simulink model "single_phase_inverter"  (R2019b)
settings: Solver=VariableStepAuto  StartTime=0.0  StopTime=0.4  RelTol=1e-3
values from neighbouring files (symbols this model uses):
  A = [-R1/L1 0 -1/L1;      0 -R2/L2 1/L2;      1/C1 -1/C1 0]    [inverter_singlephase.m]    (also in inverter_singlephase_rpi.m)
  Ae = [-R1/L1 0 -1/L1 0 0;      0 -R2/L2 1/L2 -1/L2 0;      1/C1 -1/C1 0 0 0 ... (first row only)    [inverter_singlephase.m]    (also in inverter_singlephase_rpi.m)
  B = [1/L1 0 0]'    [inverter_singlephase.m]    (also in inverter_singlephase_rpi.m)
  Be = [1/L1 0 0 0 0]'    [inverter_singlephase.m]    (also in inverter_singlephase_rpi.m)
  C = [1 0 0; 0 0 1]    [inverter_singlephase.m]    (also in inverter_singlephase_rpi.m)
  Ce = [1 0 0 0 0; 0 0 1 0 0]    [inverter_singlephase.m]    (also in inverter_singlephase_rpi.m)
  d = 3.5e-1    (= 0.35)    [inverter_singlephase.m]    (also in inverter_singlephase_rpi.m)
  E = [0 -1/L2 0]'    [inverter_singlephase.m]    (also in inverter_singlephase_rpi.m)
  K = place(A,B,[-150*2*pi,-120*2*pi,-140*2*pi])    [inverter_singlephase.m]
  L1 = 250e-6    (= 0.00025)    [inverter_singlephase.m]    (also in inverter_singlephase_rpi.m)
  L2 = 60e-6    (= 6e-05)    [inverter_singlephase.m]    (also in inverter_singlephase_rpi.m)
  Le = place(Ae',Ce',[p1,p2,p3,p4,p5])'    [inverter_singlephase.m]
  N = -inv(C(1,:)*(A-B*K)^-1*B)    [inverter_singlephase.m]
  w = 5*w0    (= 1570.79632679)    [inverter_singlephase.m]    (also in inverter_singlephase_rpi.m)
settings Model: Creator=dbagn  LastModifiedBy=dbagn

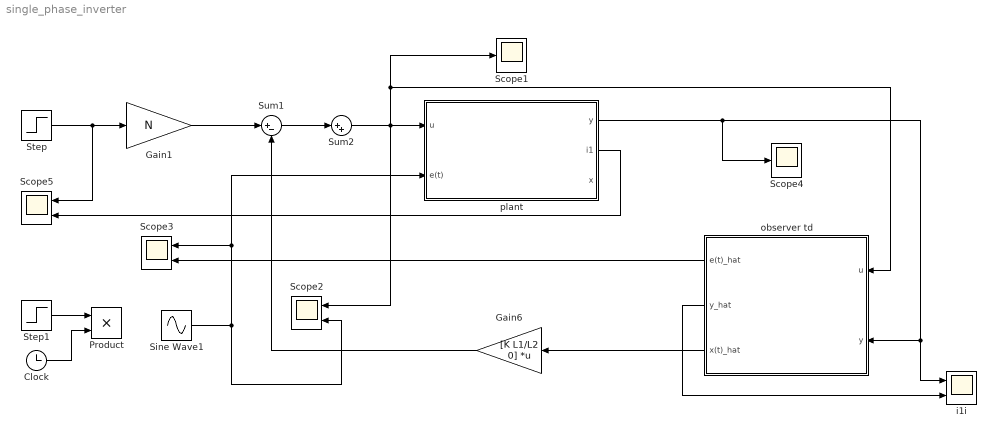
== system single_phase_inverter ==
  Clock : Clock
  Gain1 : Gain  Gain=N
  Gain6 : Gain  Gain=[K L1/L2 0]  Multiplication=Matrix(K*u)
  Product : Product
  Scope1 : Scope
  Scope2 : Scope  NumInputPorts=2
  Scope3 : Scope  NumInputPorts=2
  Scope4 : Scope
  Scope5 : Scope  NumInputPorts=2
  Sine Wave1 : Sin  Amplitude=d  Frequency=w  SampleTime=0
  Step : Step  Time=0.05  SampleTime=0
  Step1 : Step  Time=0.2  SampleTime=0
  Sum1 : Sum  Inputs=|+-
  Sum2 : Sum  Inputs=|++
  i1i : Scope  NumInputPorts=2
  observer td : Subsystem
  "plant " : Subsystem
  wires:
  observer td/2(y_hat) -> i1i/2
  "plant "/1(y) -> i1i/1, observer td/2(y), Scope4/1
  Sine Wave1/1 -> "plant "/2(e(t)), Scope3/1, Scope2/2
  observer td/1(e(t)_hat) -> Scope3/2
  "plant "/2(i1) -> Scope5/2
  Step/1 -> Gain1/1, Scope5/1
  Gain6/1 -> Sum1/2
  Gain1/1 -> Sum1/1
  Sum1/1 -> Sum2/1
  Sum2/1 -> Scope2/1, Scope1/1, observer td/1(u), "plant "/1(u)
  Step1/1 -> Product/1
  Clock/1 -> Product/2
  observer td/3(x(t)_hat) -> Gain6/1

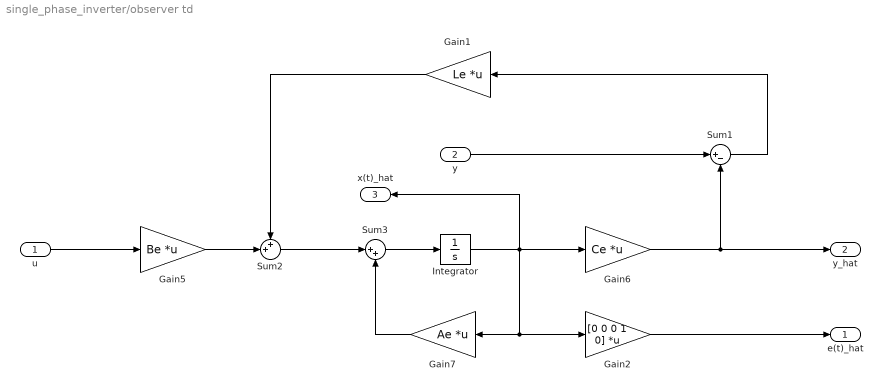
== system single_phase_inverter/observer td ==
  u : Inport
  y : Inport  Port=2
  Gain1 : Gain  Gain=Le  Multiplication=Matrix(K*u)
  Gain2 : Gain  Gain=[0 0 0 1 0]  Multiplication=Matrix(K*u)
  Gain5 : Gain  Gain=Be  Multiplication=Matrix(K*u)
  Gain6 : Gain  Gain=Ce  Multiplication=Matrix(K*u)
  Gain7 : Gain  Gain=Ae  Multiplication=Matrix(K*u)
  Integrator : Integrator
  Sum1 : Sum  Inputs=|+-
  Sum2 : Sum  Inputs=++|
  Sum3 : Sum  Inputs=|++
  e(t)_hat : Outport
  y_hat : Outport  Port=2
  x(t)_hat : Outport  Port=3
  wires:
  Sum2/1 -> Sum3/1
  Gain7/1 -> Sum3/2
  Gain6/1 -> y_hat/1, Sum1/2
  Sum1/1 -> Gain1/1
  u/1 -> Gain5/1
  Gain1/1 -> Sum2/1
  Gain5/1 -> Sum2/2
  Sum3/1 -> Integrator/1
  y/1 -> Sum1/1
  Gain2/1 -> e(t)_hat/1
  Integrator/1 -> x(t)_hat/1, Gain2/1, Gain7/1, Gain6/1

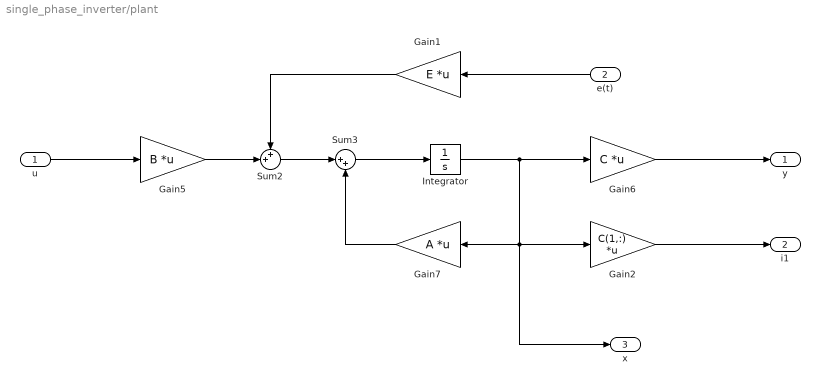
== system single_phase_inverter/plant  ==
  u : Inport
  e(t) : Inport  Port=2
  Gain1 : Gain  Gain=E  Multiplication=Matrix(K*u)
  Gain2 : Gain  Gain=C(1,:)  Multiplication=Matrix(K*u)
  Gain5 : Gain  Gain=B  Multiplication=Matrix(K*u)
  Gain6 : Gain  Gain=C  Multiplication=Matrix(K*u)
  Gain7 : Gain  Gain=A  Multiplication=Matrix(K*u)
  Integrator : Integrator
  Sum2 : Sum  Inputs=++|
  Sum3 : Sum  Inputs=|++
  y : Outport
  i1 : Outport  Port=2
  x : Outport  Port=3
  wires:
  Sum3/1 -> Integrator/1
  Gain5/1 -> Sum2/2
  Gain1/1 -> Sum2/1
  Gain7/1 -> Sum3/2
  u/1 -> Gain5/1
  Sum2/1 -> Sum3/1
  Gain6/1 -> y/1
  e(t)/1 -> Gain1/1
  Integrator/1 -> x/1, Gain2/1, Gain7/1, Gain6/1
  Gain2/1 -> i1/1
